simulink model "SF101A_MotQuadDetn"  (R2013b)
settings: Solver=FixedStepDiscrete  StartTime=0.0  StopTime=1  FixedStep=Ts  RelTol=1e-3
model workspace (MAT data in the model file):
  SLAMConfig_1_ATPP = [3707764736; 2; 1; 1; 1; 34]
values from neighbouring files (symbols this model uses):
  MotQuadDetnMotDirHysInsts = DataDict.Calibration    [SF101A_MotQuadDetn_DataDict.m]
  MOTTQCMDTOLR_MOTNWTMTR_F32 = DataDict.Constant    [SF101A_MotQuadDetn_DataDict.m]
undefined symbols (not defined in the file or in its folder): MotQuad1
libraries: simulink x5, NxtrAbslt x2, NxtrSign x2
(part 1 of 2)
settings Model: RecordCoverage=on  Creator=qzwc4r  LastModifiedBy=qzwc4r
settings DataIOCC: LimitDataPoints=off  SaveFormat=Structure  ReturnWorkspaceOutputs=on
settings OptimizationCC: BlockReduction=off  InlineParams=on  ZeroExternalMemoryAtStartup=off  ZeroInternalMemoryAtStartup=off  OptimizeModelRefInitCode=on  LifeSpan=1
settings DebuggingCC: SignalInfNanChecking=error  SignalRangeChecking=warning  UnderspecifiedInitializationDetection=Simplified  SolverPrmCheckMsg=error  InheritedTsInSrcMsg=error  DiscreteInheritContinuousMsg=error  SingleTaskRateTransMsg=error  TasksWithSamePriorityMsg=error  SigSpecEnsureSampleTimeMsg=error  CheckMatrixSingularityMsg=error  IntegerOverflowMsg=error  ParameterUnderflowMsg=error  ParameterPrecisionLossMsg=error  ParameterTunabilityLossMsg=error  FixptConstUnderflowMsg=warning  FixptConstOverflowMsg=warning  VectorMatrixConversionMsg=error  SignalLabelMismatchMsg=error  UnconnectedInputMsg=error  UnconnectedOutputMsg=error  UnconnectedLineMsg=error  SFcnCompatibilityMsg=error  UniqueDataStoreMsg=warning  BusObjectLabelMismatch=error  RootOutportRequireBusObject=error  AssertControl=DisableAll  ModelReferenceIOMsg=error  ModelReferenceVersionMismatchMessage=warning  ModelReferenceIOMismatchMessage=error  ModelReferenceCSMismatchMessage=warning  ModelReferenceDataLoggingMessage=error  StateNameClashWarn=warning  StrictBusMsg=ErrorOnBusTreatedAsVector  NonBusSignalsTreatedAsBus=error  SFUnexpectedBacktrackingDiag=error  SFInvalidInputDataAccessInChartInitDiag=error  SFNoUnconditionalDefaultTransitionDiag=error  SFTransitionOutsideNaturalParentDiag=error  SFUnconditionalTransitionShadowingDiag=error  SFUndirectedBroadcastEventsDiag=error
settings ModelReferenceCC: ModelReferenceNumInstancesAllowed=Single
settings RTWCC: SystemTargetFile=autosar.tlc  GenCodeOnly=on  TemplateMakefile=ert_default_tmf  Description=AUTOSAR  GenerateReport=on  ProcessScript=autosar_make_rtw_hook  LaunchReport=on
settings CodeAppCC: GenerateComments=off  IgnoreCustomStorageClasses=off  CustomSymbolStrType=$N$R$M  CustomSymbolStrBlkIO=$N$M  SimulinkBlockComments=off
settings STFCustomTargetCC: ParMdlRefBuildCompliant=on  CompOptLevelCompliant=on  IncludeMdlTerminateFcn=off  CombineOutputUpdateFcns=on  SuppressErrorStatus=on  ERTFirstTimeCompliant=on  ERTCustomFileBanners=on  SupportNonFinite=off  SupportComplex=off  SupportContinuousTime=off  SupportNonInlinedSFcns=off  MATLABClassNameForMDSCustomization=Simulink.SoftwareTarget.ERTCustomization  AutosarCompliant=on  GRTInterface=off  SystemTargetFile=autosar.tlc
settings ERTTargetCC: CodeReplacementLibrary=ANSI_C  ConcurrentExecutionCompliant=off  IncludeMdlTerminateFcn=off  SuppressErrorStatus=on  SupportNonFinite=off  SupportComplex=off  ModelStepFunctionPrototypeControlCompliant=off  CPPClassGenCompliant=off  AutosarCompliant=on  InlinedParameterPlacement=NonHierarchical  ERTCustomFileTemplate=example_file_process.tlc  EnableUserReplacementTypes=on

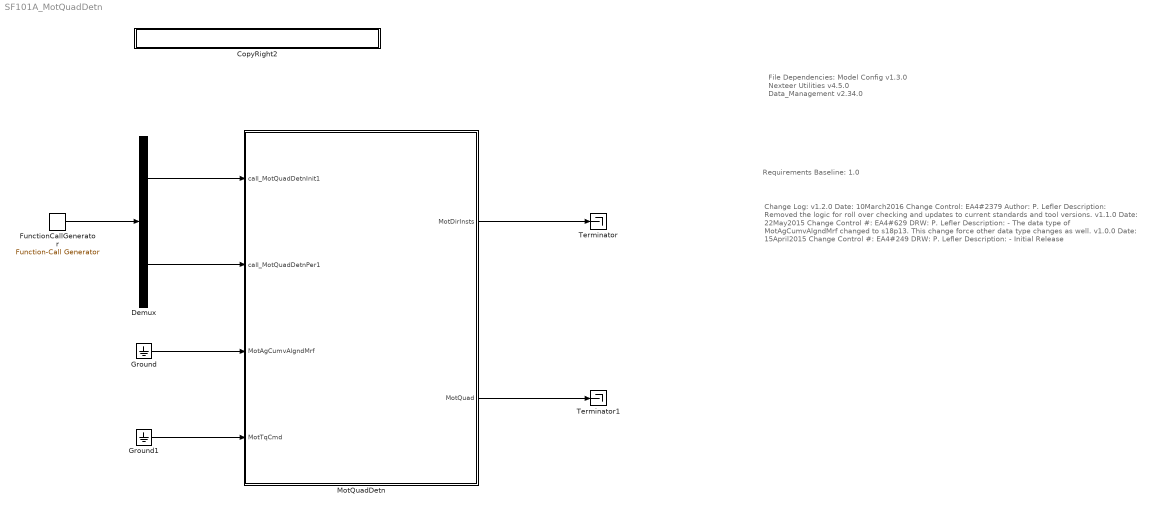
== system SF101A_MotQuadDetn ==
  note: File Dependencies:
      |
      | Model Config v1.3.0
      | Nexteer Utilities v4.5.0
      | Data_Management v2.34.0
  note: Requirements Baseline: 1.0
  note: Change Log:
      |
      | v1.2.0
      | Date: 10March2016
      | Change Control: EA4#2379
      | Author: P. Lefler
      | Description:
      | Removed the logic for roll over checking and updates to current standards and tool versions.
      |
      | v1.1.0
      | Date: 22May2015
      | Change Control #: EA4#629
      | DRW: P. Lefler
      | Description:
      | - The data type of MotAgCumvAlgndMrf changed to s18p13.
      |   This change force other data type changes as well.
      |
      | v1.0.0
      | Date: 15April2015
      | Change Control #: EA4#249
      | DRW: P. Lefler
      | Description:
      | - Initial Release
  CopyRight2 : Subsystem  Description=|  mask(Copyright Information){none=on}
      | Copyright info block.                                               
      |                                                                     
      | Place copyright information at the top of every subsystem in design.
      mask prompts: none "No parameters"
      mask help: Place copyright information at the top of every subsystem in design.
      mask Display:
      | NxtrConf = 'Nexteer Confidential';
      | 
      | sys = bdroot; %handle for the current model ("system")
      | first = get_param(sys,'Created');
      | if(isempty(first))
      |     first = datestr(now,'yyyy');
      | else
      |     first = first(end-3:end);  %year is last four digits
      | end
      | 
      | last = get_param(sys,'LastModifiedDate');
      | if isempty(last)
      |     last = datestr(now,'yyyy');
      | else
      |     last = last(end-3:end);
      | end
      | 
      | if strcmp(first,last)
      |     fprintf('%s -- Copyright %s Nexteer',NxtrConf,first)
      | else
      |     fprintf('%s -- %s%s- %s Nexteer',NxtrConf,char(169),first,last)
      | end
  Demux : Demux  Outputs=2
  FunctionCallGenerator : simulink/Ports & Subsystems/Function-Call Generator  RequirementInfo="{'linktype_rmi_doors' '0000bb40 (/E-STEER Core/SubSystem Specifications/Application Functions/SF99/SF101A Motor Quadrant Detection)' '#SF101A_63' 'true' 'REQ:  SF101A_63' '' } %GIDa_ba4b940a_c476_4c12_9873_433c070b2edb"  sample_time=0.002  numberOfIterations=1
  Ground : Ground
  Ground1 : Ground
  MotQuadDetn : Subsystem
  Terminator : Terminator
  Terminator1 : Terminator
  wires:
  Demux/1 -> MotQuadDetn/1(call_MotQuadDetnInit1)
  Demux/2 -> MotQuadDetn/2(call_MotQuadDetnPer1)
  FunctionCallGenerator/1 -> Demux/1
  Ground/1 -> MotQuadDetn/3(MotAgCumvAlgndMrf)
  MotQuadDetn/1(MotDirInsts) -> Terminator/1
  MotQuadDetn/2(MotQuad) -> Terminator1/1
  Ground1/1 -> MotQuadDetn/4(MotTqCmd)

== system SF101A_MotQuadDetn/CopyRight2 ==

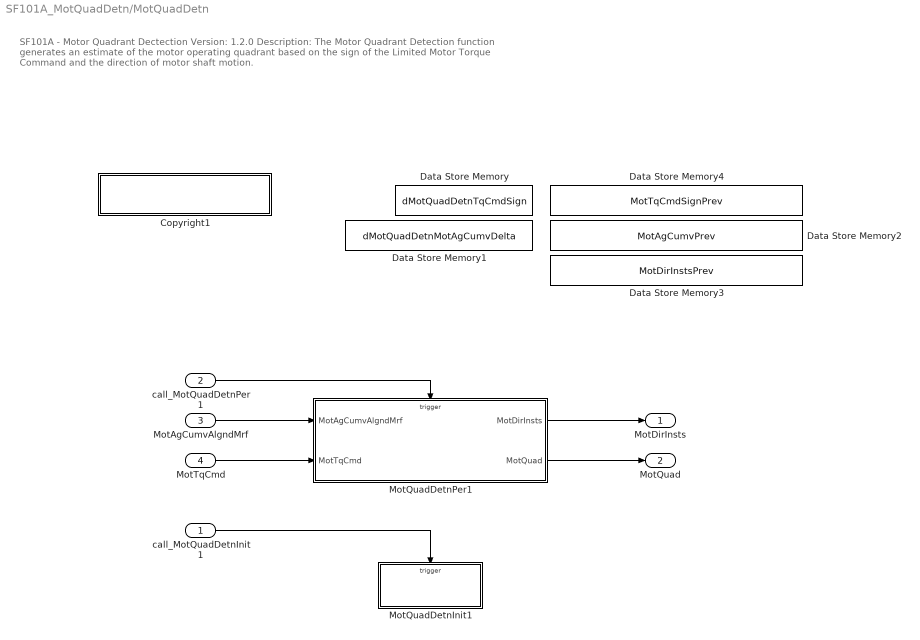
== system SF101A_MotQuadDetn/MotQuadDetn ==
  note: SF101A - Motor Quadrant Dectection
      | Version: 1.2.0
      | Description:
      | The Motor Quadrant Detection function generates an estimate of the motor operating quadrant based on the sign of the Limited Motor Torque Command and the direction of motor shaft motion.
  call_MotQuadDetnInit1 : Inport
  call_MotQuadDetnPer1 : Inport  Port=2
  MotAgCumvAlgndMrf : Inport  RequirementInfo="{'linktype_rmi_doors' '0000bb40 (/E-STEER Core/SubSystem Specifications/Application Functions/SF99/SF101A Motor Quadrant Detection)' '#SF101A_27' 'true' 'REQ:  SF101A_27' '' } %GIDa_ce1f5992_a30b_4fb4_84ed_8bc9c57286df"  Port=3  OutDataTypeStr=int32  PortDimensions=1
  MotTqCmd : Inport  RequirementInfo="{'linktype_rmi_doors' '0000bb40 (/E-STEER Core/SubSystem Specifications/Application Functions/SF99/SF101A Motor Quadrant Detection)' '#SF101A_38' 'true' 'REQ:  SF101A_38' '' } %GIDa_55ad6957_dc0e_47dc_876d_670590d48796"  Port=4  OutDataTypeStr=single  PortDimensions=1
  Copyright1 : Subsystem  Description=|  mask(Copyright Information){none=on}
      | Copyright info block.                                               
      |                                                                     
      | Place copyright information at the top of every subsystem in design.
      mask prompts: none "No parameters"
      mask help: Place copyright information at the top of every subsystem in design.
      mask Display:
      | NxtrConf = 'Nexteer Confidential';
      | 
      | sys = bdroot; %handle for the current model ("system")
      | first = get_param(sys,'Created');
      | if(isempty(first))
      |     first = datestr(now,'yyyy');
      | else
      |     first = first(end-3:end);  %year is last four digits
      | end
      | 
      | last = get_param(sys,'LastModifiedDate');
      | if isempty(last)
      |     last = datestr(now,'yyyy');
      | else
      |     last = last(end-3:end);
      | end
      | 
      | if strcmp(first,last)
      |     fprintf('%s\nCopyright  %s Nexteer',NxtrConf,first);
      | else
      |     fprintf('%s\n%s%s-%s Nexteer',NxtrConf,char(169),first,last);
      | end
  Data Store Memory : DataStoreMemory  DataStoreName=dMotQuadDetnTqCmdSign  StateMustResolveToSignalObject=on
  Data Store Memory1 : DataStoreMemory  DataStoreName=dMotQuadDetnMotAgCumvDelta  StateMustResolveToSignalObject=on
  Data Store Memory2 : DataStoreMemory  DataStoreName=MotAgCumvPrev  StateMustResolveToSignalObject=on
  Data Store Memory3 : DataStoreMemory  DataStoreName=MotDirInstsPrev  StateMustResolveToSignalObject=on
  Data Store Memory4 : DataStoreMemory  DataStoreName=MotTqCmdSignPrev  StateMustResolveToSignalObject=on
  MotQuadDetnInit1 : Subsystem  TreatAsAtomicUnit=on
  MotQuadDetnPer1 : Subsystem
  MotDirInsts : Outport  RequirementInfo="{'linktype_rmi_doors' '0000bb40 (/E-STEER Core/SubSystem Specifications/Application Functions/SF99/SF101A Motor Quadrant Detection)' '#SF101A_28' 'true' 'REQ:  SF101A_28' '' } %GIDa_c93875f8_cc59_405f_b59a_8f59cf744667"  OutDataTypeStr=int8  PortDimensions=1
  MotQuad : Outport  RequirementInfo="{'linktype_rmi_doors' '0000bb40 (/E-STEER Core/SubSystem Specifications/Application Functions/SF99/SF101A Motor Quadrant Detection)' '#SF101A_39' 'true' 'REQ:  SF101A_39' '' } %GIDa_9a3fad06_e616_455b_a302_26a30b94c3d7"  Port=2  OutDataTypeStr=Enum: MotQuad1  PortDimensions=1
  wires:
  MotQuadDetnPer1/2(MotQuad) -> MotQuad/1
  MotQuadDetnPer1/1(MotDirInsts) -> MotDirInsts/1
  MotTqCmd/1 -> MotQuadDetnPer1/2(MotTqCmd)
  MotAgCumvAlgndMrf/1 -> MotQuadDetnPer1/1(MotAgCumvAlgndMrf)
  call_MotQuadDetnPer1/1 -> MotQuadDetnPer1/Trigger
  call_MotQuadDetnInit1/1 -> MotQuadDetnInit1/Trigger

== system SF101A_MotQuadDetn/MotQuadDetn/Copyright1 ==

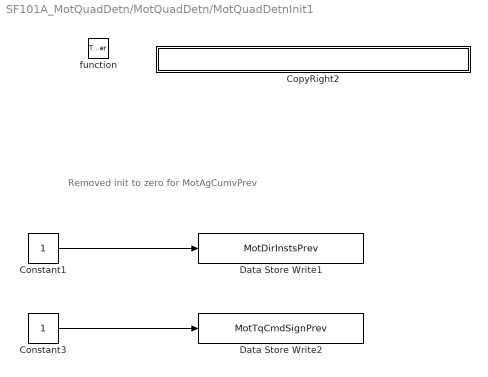
== system SF101A_MotQuadDetn/MotQuadDetn/MotQuadDetnInit1 ==
  note: Removed init to zero for MotAgCumvPrev
  function : TriggerPort  TriggerType=function-call
  Constant1 : Constant  RequirementInfo="{'linktype_rmi_doors' '0000bb40 (/E-STEER Core/SubSystem Specifications/Application Functions/SF99/SF101A Motor Quadrant Detection)' '#SF101A_49' 'true' 'REQ:  SF101A_49' '' } %GIDa_5d2ddbe5_3095_4ce2_977e_d4f70d111454"  OutDataTypeStr=int8
  Constant3 : Constant  RequirementInfo="{'linktype_rmi_doors' '0000bb40 (/E-STEER Core/SubSystem Specifications/Application Functions/SF99/SF101A Motor Quadrant Detection)' '#SF101A_55' 'true' 'REQ:  SF101A_55' '' } %GIDa_37157d88_6289_46d7_8e4c_5fdd13e4fc16"  OutDataTypeStr=int8
  CopyRight2 : Subsystem  Description=|  mask(Copyright Information){none=on}
      | Copyright info block.                                               
      |                                                                     
      | Place copyright information at the top of every subsystem in design.
      mask prompts: none "No parameters"
      mask help: Place copyright information at the top of every subsystem in design.
      mask Display:
      | NxtrConf = 'Nexteer Confidential';
      | 
      | sys = bdroot; %handle for the current model ("system")
      | first = get_param(sys,'Created');
      | if(isempty(first))
      |     first = datestr(now,'yyyy');
      | else
      |     first = first(end-3:end);  %year is last four digits
      | end
      | 
      | last = get_param(sys,'LastModifiedDate');
      | if isempty(last)
      |     last = datestr(now,'yyyy');
      | else
      |     last = last(end-3:end);
      | end
      | 
      | if strcmp(first,last)
      |     fprintf('%s -- Copyright %s Nexteer',NxtrConf,first)
      | else
      |     fprintf('%s -- %s%s- %s Nexteer',NxtrConf,char(169),first,last)
      | end
  Data Store Write1 : DataStoreWrite  RequirementInfo="{'linktype_rmi_doors' '0000bb40 (/E-STEER Core/SubSystem Specifications/Application Functions/SF99/SF101A Motor Quadrant Detection)' '#SF101A_49' 'true' 'REQ:  SF101A_49' '' } %GIDa_33825ee6_1fe0_4111_9478_8621974325d7"  DataStoreName=MotDirInstsPrev
  Data Store Write2 : DataStoreWrite  RequirementInfo="{'linktype_rmi_doors' '0000bb40 (/E-STEER Core/SubSystem Specifications/Application Functions/SF99/SF101A Motor Quadrant Detection)' '#SF101A_55' 'true' 'REQ:  SF101A_55' '' } %GIDa_0551e2d3_8a0f_49e4_ae02_6b9d57023870"  DataStoreName=MotTqCmdSignPrev
  wires:
  Constant1/1 -> Data Store Write1/1
  Constant3/1 -> Data Store Write2/1

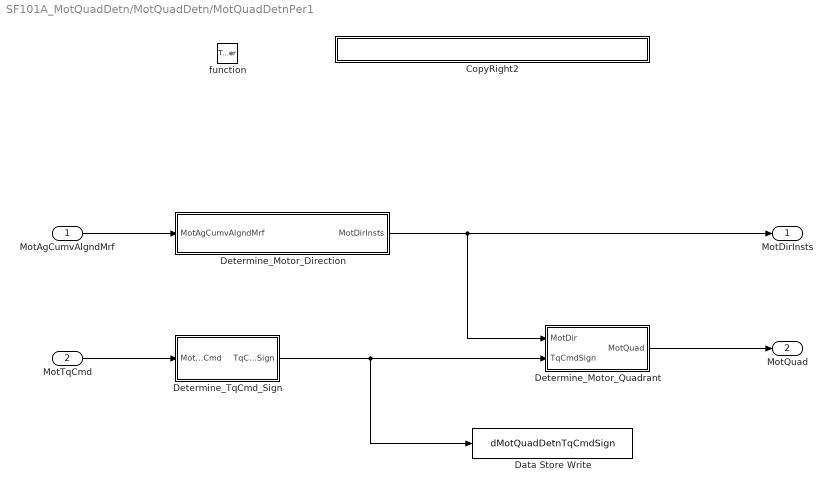
== system SF101A_MotQuadDetn/MotQuadDetn/MotQuadDetnPer1 ==
  MotAgCumvAlgndMrf : Inport  OutDataTypeStr=int32  PortDimensions=1
  MotTqCmd : Inport  Port=2  OutDataTypeStr=single  PortDimensions=1
  function : TriggerPort  TriggerType=function-call  PortDimensions=1
  CopyRight2 : Subsystem  Description=|  mask(Copyright Information){none=on}
      | Copyright info block.                                               
      |                                                                     
      | Place copyright information at the top of every subsystem in design.
      mask prompts: none "No parameters"
      mask help: Place copyright information at the top of every subsystem in design.
      mask Display:
      | NxtrConf = 'Nexteer Confidential';
      | 
      | sys = bdroot; %handle for the current model ("system")
      | first = get_param(sys,'Created');
      | if(isempty(first))
      |     first = datestr(now,'yyyy');
      | else
      |     first = first(end-3:end);  %year is last four digits
      | end
      | 
      | last = get_param(sys,'LastModifiedDate');
      | if isempty(last)
      |     last = datestr(now,'yyyy');
      | else
      |     last = last(end-3:end);
      | end
      | 
      | if strcmp(first,last)
      |     fprintf('%s -- Copyright %s Nexteer',NxtrConf,first)
      | else
      |     fprintf('%s -- %s%s- %s Nexteer',NxtrConf,char(169),first,last)
      | end
  Data Store Write : DataStoreWrite  DataStoreName=dMotQuadDetnTqCmdSign
  Determine_Motor_Direction : Subsystem  TreatAsAtomicUnit=on
  Determine_Motor_Quadrant : Subsystem  RequirementInfo="{'linktype_rmi_doors' '0000bb40 (/E-STEER Core/SubSystem Specifications/Application Functions/SF99/SF101A Motor Quadrant Detection)' '#SF101A_53' 'true' 'REQ:  SF101A_53' '' } %GIDa_02fb40bd_96d0_49ba_b5f0_97be253398e5"  TreatAsAtomicUnit=on
  Determine_TqCmd_Sign : Subsystem  RequirementInfo="{'linktype_rmi_doors' '0000bb40 (/E-STEER Core/SubSystem Specifications/Application Functions/SF99/SF101A Motor Quadrant Detection)' '#SF101A_51' 'true' 'REQ:  SF101A_51' '' } %GIDa_eb9f9e8f_fed9_4594_8edb_e305cda2f43b"  TreatAsAtomicUnit=on
  MotDirInsts : Outport  OutDataTypeStr=int8  PortDimensions=1
  MotQuad : Outport  Port=2  OutDataTypeStr=Enum: MotQuad1  PortDimensions=1
  wires:
  MotAgCumvAlgndMrf/1 -> Determine_Motor_Direction/1(MotAgCumvAlgndMrf)
  MotTqCmd/1 -> Determine_TqCmd_Sign/1(MotTqCmd)
  Determine_TqCmd_Sign/1(TqCmdSign) -> Data Store Write/1, Determine_Motor_Quadrant/2(TqCmdSign)
  Determine_Motor_Quadrant/1(MotQuad) -> MotQuad/1
  Determine_Motor_Direction/1(MotDirInsts) -> MotDirInsts/1, Determine_Motor_Quadrant/1(MotDir)

== system SF101A_MotQuadDetn/MotQuadDetn/MotQuadDetnInit1/CopyRight2 ==

== system SF101A_MotQuadDetn/MotQuadDetn/MotQuadDetnPer1/CopyRight2 ==

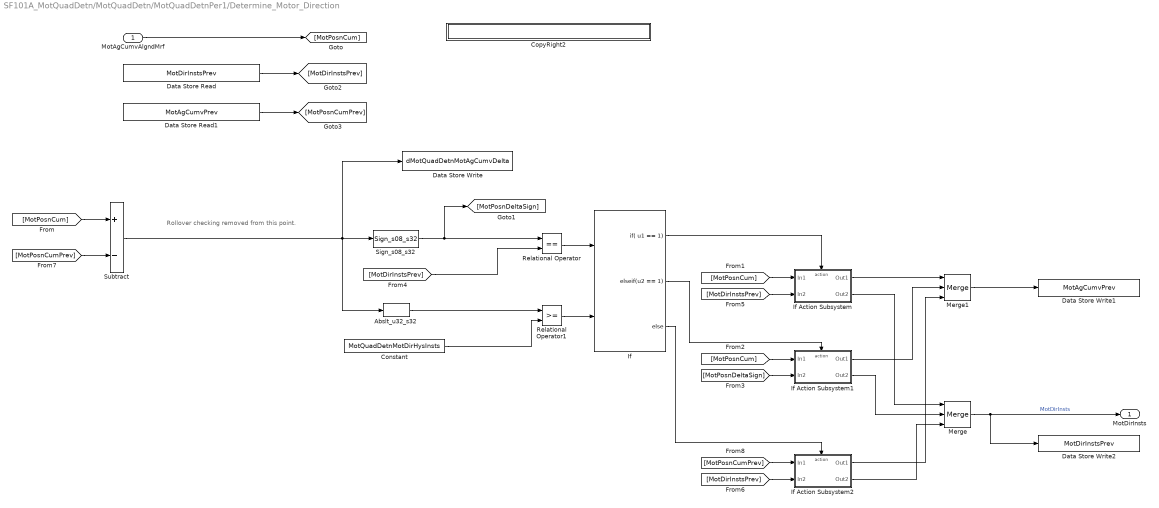
== system SF101A_MotQuadDetn/MotQuadDetn/MotQuadDetnPer1/Determine_Motor_Direction ==
  note: Rollover checking removed from this point.
  MotAgCumvAlgndMrf : Inport  RequirementInfo="{'linktype_rmi_doors' '0000bb40 (/E-STEER Core/SubSystem Specifications/Application Functions/SF99/SF101A Motor Quadrant Detection)' '#SF101A_46' 'true' 'REQ:  SF101A_46' '' ; 'linktype_rmi_doors' '0000bb40 (/E-STEER Core/SubSystem Specifications/Application Functions/SF99/SF101A Motor Quadrant Detection)' '#SF101A_44' 'true' 'REQ:  SF101A_44' '' } %GIDa_33168858_7d05_4f18_8f4c_06695088646f"
  Abslt_u32_s32 : NxtrAbslt/Abslt_u32_s32  RequirementInfo="{'linktype_rmi_doors' '0000bb40 (/E-STEER Core/SubSystem Specifications/Application Functions/SF99/SF101A Motor Quadrant Detection)' '#SF101A_47' 'true' 'REQ:  SF101A_47' '' } %GIDa_46c42c72_ca25_40ef_8955_407cadf23955"  SFunctionSpec=uint32 y1 = Abslt_u32_s32( int32 u1)
      settings: AttributesFormatString=%<Name>
  Constant : Constant  RequirementInfo="{'linktype_rmi_doors' '0000bb40 (/E-STEER Core/SubSystem Specifications/Application Functions/SF99/SF101A Motor Quadrant Detection)' '#SF101A_47' 'true' 'REQ:  SF101A_47' '' } %GIDa_7af5e37b_1e32_4084_9345_8c4ddd29f877"  Value=MotQuadDetnMotDirHysInsts
  CopyRight2 : Subsystem  Description=|  mask(Copyright Information){none=on}
      | Copyright info block.                                               
      |                                                                     
      | Place copyright information at the top of every subsystem in design.
      mask prompts: none "No parameters"
      mask help: Place copyright information at the top of every subsystem in design.
      mask Display:
      | NxtrConf = 'Nexteer Confidential';
      | 
      | sys = bdroot; %handle for the current model ("system")
      | first = get_param(sys,'Created');
      | if(isempty(first))
      |     first = datestr(now,'yyyy');
      | else
      |     first = first(end-3:end);  %year is last four digits
      | end
      | 
      | last = get_param(sys,'LastModifiedDate');
      | if isempty(last)
      |     last = datestr(now,'yyyy');
      | else
      |     last = last(end-3:end);
      | end
      | 
      | if strcmp(first,last)
      |     fprintf('%s -- Copyright %s Nexteer',NxtrConf,first)
      | else
      |     fprintf('%s -- %s%s- %s Nexteer',NxtrConf,char(169),first,last)
      | end
  Data Store Read : DataStoreRead  DataStoreName=MotDirInstsPrev
  Data Store Read1 : DataStoreRead  RequirementInfo="{'linktype_rmi_doors' '0000bb40 (/E-STEER Core/SubSystem Specifications/Application Functions/SF99/SF101A Motor Quadrant Detection)' '#SF101A_46' 'true' 'REQ:  SF101A_46' '' ; 'linktype_rmi_doors' '0000bb40 (/E-STEER Core/SubSystem Specifications/Application Functions/SF99/SF101A Motor Quadrant Detection)' '#SF101A_44' 'true' 'REQ:  SF101A_44' '' } %GIDa_269066c3_13eb_447a_8e55_95ebd7583ac8"  DataStoreName=MotAgCumvPrev
  Data Store Write : DataStoreWrite  DataStoreName=dMotQuadDetnMotAgCumvDelta
  Data Store Write1 : DataStoreWrite  RequirementInfo="{'linktype_rmi_doors' '0000bb40 (/E-STEER Core/SubSystem Specifications/Application Functions/SF99/SF101A Motor Quadrant Detection)' '#SF101A_46' 'true' 'REQ:  SF101A_46' '' ; 'linktype_rmi_doors' '0000bb40 (/E-STEER Core/SubSystem Specifications/Application Functions/SF99/SF101A Motor Quadrant Detection)' '#SF101A_44' 'true' 'REQ:  SF101A_44' '' } %GIDa_9bff677e_e394_40d8_a69c_2132827397bf"  DataStoreName=MotAgCumvPrev
  Data Store Write2 : DataStoreWrite  DataStoreName=MotDirInstsPrev
  If : If  NumInputs=2  IfExpression=u1 == 1  ElseIfExpressions=u2 == 1
  If Action Subsystem : Subsystem  TreatAsAtomicUnit=on
      settings: RTWSystemCode=Inline
  If Action Subsystem1 : Subsystem  TreatAsAtomicUnit=on
      settings: RTWSystemCode=Inline
  If Action Subsystem2 : Subsystem  TreatAsAtomicUnit=on
      settings: RTWSystemCode=Inline
  Merge : Merge  Inputs=3
  Merge1 : Merge  Inputs=3
  Relational Operator : RelationalOperator  Operator===  OutDataTypeStr=boolean
  Relational Operator1 : RelationalOperator  OutDataTypeStr=boolean
  Sign_s08_s32 : NxtrSign/Sign_s08_s32  RequirementInfo="{'linktype_rmi_doors' '0000bb40 (/E-STEER Core/SubSystem Specifications/Application Functions/SF99/SF101A Motor Quadrant Detection)' '#SF101A_44' 'true' 'REQ:  SF101A_44' '' ; 'linktype_rmi_doors' '0000bb40 (/E-STEER Core/SubSystem Specifications/Application Functions/SF99/SF101A Motor Quadrant Detection)' '#SF101A_57' 'true' 'REQ:  SF101A_57' '' } %GIDa_4174577c_cdf4_4d25_8cc3_032965890b4a"  SFunctionSpec=int8 y1 = Sign_s08_s32( int32 u1)
  Subtract : Sum  RequirementInfo="{'linktype_rmi_doors' '0000bb40 (/E-STEER Core/SubSystem Specifications/Application Functions/SF99/SF101A Motor Quadrant Detection)' '#SF101A_46' 'true' 'REQ:  SF101A_46' '' ; 'linktype_rmi_doors' '0000bb40 (/E-STEER Core/SubSystem Specifications/Application Functions/SF99/SF101A Motor Quadrant Detection)' '#SF101A_44' 'true' 'REQ:  SF101A_44' '' } %GIDa_5fce257d_7301_4941_b31f_c4ddb6e8cb64"  Inputs=+-
  MotDirInsts : Outport
  wires:
  [MotPosnCumPrev] -> Subtract/2
  Sign_s08_s32/1 -> Relational Operator/1, [MotPosnDeltaSign]
  If/1 -> If Action Subsystem/Action
  If/2 -> If Action Subsystem1/Action
  MotAgCumvAlgndMrf/1 -> [MotPosnCum]
  [MotPosnCum] -> Subtract/1
  [MotPosnCum] -> If Action Subsystem/1(In1)
  [MotPosnCum] -> If Action Subsystem1/1(In1)
  [MotPosnDeltaSign] -> If Action Subsystem1/2(In2)
  [MotDirInstsPrev] -> Relational Operator/2
  [MotPosnCumPrev] -> If Action Subsystem2/1(In1)
  If/3 -> If Action Subsystem2/Action
  If Action Subsystem2/2(Out2) -> Merge/3
  If Action Subsystem1/2(Out2) -> Merge/2
  If Action Subsystem/2(Out2) -> Merge/1
  Merge/1 -> Data Store Write2/1, MotDirInsts/1  "MotDirInsts"
  If Action Subsystem/1(Out1) -> Merge1/1
  If Action Subsystem1/1(Out1) -> Merge1/2
  If Action Subsystem2/1(Out1) -> Merge1/3
  Merge1/1 -> Data Store Write1/1
  Subtract/1 -> Data Store Write/1, Abslt_u32_s32/1, Sign_s08_s32/1
  [MotDirInstsPrev] -> If Action Subsystem/2(In2)
  [MotDirInstsPrev] -> If Action Subsystem2/2(In2)
  Data Store Read/1 -> [MotDirInstsPrev]
  Data Store Read1/1 -> [MotPosnCumPrev]
  Constant/1 -> Relational Operator1/2
  Abslt_u32_s32/1 -> Relational Operator1/1
  Relational Operator1/1 -> If/2
  Relational Operator/1 -> If/1

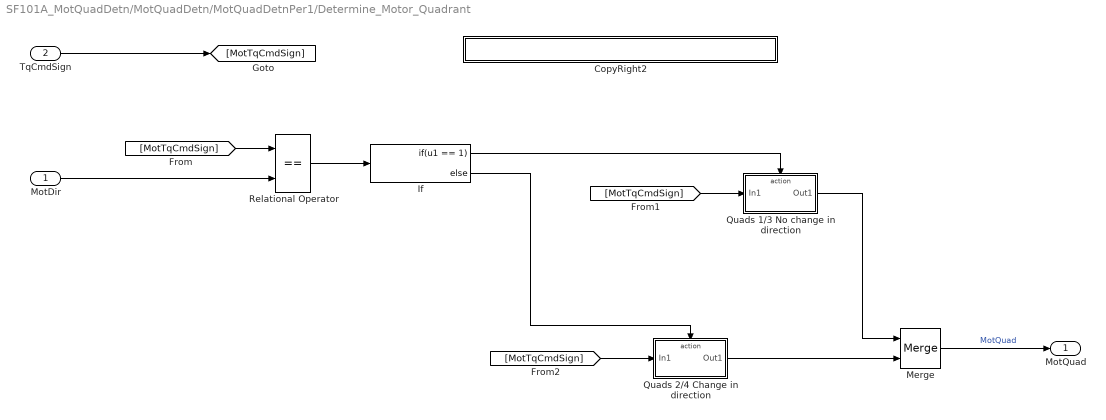
== system SF101A_MotQuadDetn/MotQuadDetn/MotQuadDetnPer1/Determine_Motor_Quadrant ==
  MotDir : Inport
  TqCmdSign : Inport  Port=2
  CopyRight2 : Subsystem  Description=|  mask(Copyright Information){none=on}
      | Copyright info block.                                               
      |                                                                     
      | Place copyright information at the top of every subsystem in design.
      mask prompts: none "No parameters"
      mask help: Place copyright information at the top of every subsystem in design.
      mask Display:
      | NxtrConf = 'Nexteer Confidential';
      | 
      | sys = bdroot; %handle for the current model ("system")
      | first = get_param(sys,'Created');
      | if(isempty(first))
      |     first = datestr(now,'yyyy');
      | else
      |     first = first(end-3:end);  %year is last four digits
      | end
      | 
      | last = get_param(sys,'LastModifiedDate');
      | if isempty(last)
      |     last = datestr(now,'yyyy');
      | else
      |     last = last(end-3:end);
      | end
      | 
      | if strcmp(first,last)
      |     fprintf('%s -- Copyright %s Nexteer',NxtrConf,first)
      | else
      |     fprintf('%s -- %s%s- %s Nexteer',NxtrConf,char(169),first,last)
      | end
  If : If  RequirementInfo="{'linktype_rmi_doors' '0000bb40 (/E-STEER Core/SubSystem Specifications/Application Functions/SF99/SF101A Motor Quadrant Detection)' '#SF101A_54' 'true' 'REQ:  SF101A_54' '' } %GIDa_7ecc17ff_8f5e_4b14_8da8_ae67d5ff9ccc"  IfExpression=u1 == 1
  Merge : Merge  RequirementInfo="{'linktype_rmi_doors' '0000bb40 (/E-STEER Core/SubSystem Specifications/Application Functions/SF99/SF101A Motor Quadrant Detection)' '#SF101A_54' 'true' 'REQ:  SF101A_54' '' } %GIDa_c93a8099_e8e5_4c0b_987a_8154384b51c5"
  Quads 1/3 No change in direction : Subsystem  RequirementInfo="{'linktype_rmi_doors' '0000bb40 (/E-STEER Core/SubSystem Specifications/Application Functions/SF99/SF101A Motor Quadrant Detection)' '#SF101A_54' 'true' 'REQ:  SF101A_54' '' } %GIDa_1c85d6fb_bcbe_4ead_8f35_8795b5e2ff89"  TreatAsAtomicUnit=on
      settings: RTWSystemCode=Inline
  Quads 2/4 Change in direction : Subsystem  RequirementInfo="{'linktype_rmi_doors' '0000bb40 (/E-STEER Core/SubSystem Specifications/Application Functions/SF99/SF101A Motor Quadrant Detection)' '#SF101A_54' 'true' 'REQ:  SF101A_54' '' } %GIDa_e2a8a1e9_6f7b_4770_8502_8c1a72a8d8f8"  TreatAsAtomicUnit=on
      settings: RTWSystemCode=Inline
  Relational Operator : RelationalOperator  RequirementInfo="{'linktype_rmi_doors' '0000bb40 (/E-STEER Core/SubSystem Specifications/Application Functions/SF99/SF101A Motor Quadrant Detection)' '#SF101A_54' 'true' 'REQ:  SF101A_54' '' } %GIDa_b4a959e3_569f_4f7a_bb72_55e412dce501"  Operator===  OutDataTypeStr=boolean
  MotQuad : Outport
  wires:
  Relational Operator/1 -> If/1
  If/1 -> Quads 1/3 No change in direction/Action
  If/2 -> Quads 2/4 Change in direction/Action
  [MotTqCmdSign] -> Relational Operator/1
  [MotTqCmdSign] -> Quads 1/3 No change in direction/1(In1)
  [MotTqCmdSign] -> Quads 2/4 Change in direction/1(In1)
  Quads 2/4 Change in direction/1(Out1) -> Merge/2
  Quads 1/3 No change in direction/1(Out1) -> Merge/1
  Merge/1 -> MotQuad/1  "MotQuad"
  MotDir/1 -> Relational Operator/2
  TqCmdSign/1 -> [MotTqCmdSign]

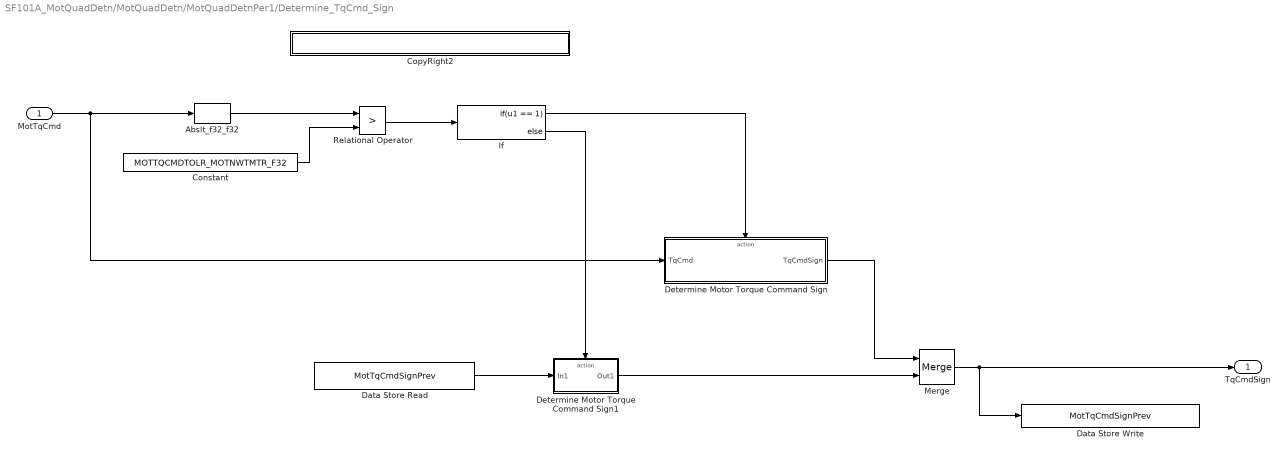
== system SF101A_MotQuadDetn/MotQuadDetn/MotQuadDetnPer1/Determine_TqCmd_Sign ==
  MotTqCmd : Inport
  Abslt_f32_f32 : NxtrAbslt/Abslt_f32_f32  RequirementInfo="{'linktype_rmi_doors' '0000bb40 (/E-STEER Core/SubSystem Specifications/Application Functions/SF99/SF101A Motor Quadrant Detection)' '#SF101A_51' 'true' 'REQ:  SF101A_51' '' ; 'linktype_rmi_doors' '0000bb40 (/E-STEER Core/SubSystem Specifications/Application Functions/SF99/SF101A Motor Quadrant Detection)' '#SF101A_52' 'true' 'REQ:  SF101A_52' '' } %GIDa_f90e4f93_60c7_4e66_b13a_2d2178dfe548"  SFunctionSpec=single y1 = Abslt_f32_f32(single u1)
      settings: AttributesFormatString=%<Name>
  Constant : Constant  RequirementInfo="{'linktype_rmi_doors' '0000bb40 (/E-STEER Core/SubSystem Specifications/Application Functions/SF99/SF101A Motor Quadrant Detection)' '#SF101A_51' 'true' 'REQ:  SF101A_51' '' ; 'linktype_rmi_doors' '0000bb40 (/E-STEER Core/SubSystem Specifications/Application Functions/SF99/SF101A Motor Quadrant Detection)' '#SF101A_52' 'true' 'REQ:  SF101A_52' '' } %GIDa_e193f212_06fe_40ea_a857_e74bcfb91209"  Value=MOTTQCMDTOLR_MOTNWTMTR_F32
  CopyRight2 : Subsystem  Description=|  mask(Copyright Information){none=on}
      | Copyright info block.                                               
      |                                                                     
      | Place copyright information at the top of every subsystem in design.
      mask prompts: none "No parameters"
      mask help: Place copyright information at the top of every subsystem in design.
      mask Display:
      | NxtrConf = 'Nexteer Confidential';
      | 
      | sys = bdroot; %handle for the current model ("system")
      | first = get_param(sys,'Created');
      | if(isempty(first))
      |     first = datestr(now,'yyyy');
      | else
      |     first = first(end-3:end);  %year is last four digits
      | end
      | 
      | last = get_param(sys,'LastModifiedDate');
      | if isempty(last)
      |     last = datestr(now,'yyyy');
      | else
      |     last = last(end-3:end);
      | end
      | 
      | if strcmp(first,last)
      |     fprintf('%s -- Copyright %s Nexteer',NxtrConf,first)
      | else
      |     fprintf('%s -- %s%s- %s Nexteer',NxtrConf,char(169),first,last)
      | end
  Data Store Read : DataStoreRead  RequirementInfo="{'linktype_rmi_doors' '0000bb40 (/E-STEER Core/SubSystem Specifications/Application Functions/SF99/SF101A Motor Quadrant Detection)' '#SF101A_51' 'true' 'REQ:  SF101A_51' '' ; 'linktype_rmi_doors' '0000bb40 (/E-STEER Core/SubSystem Specifications/Application Functions/SF99/SF101A Motor Quadrant Detection)' '#SF101A_52' 'true' 'REQ:  SF101A_52' '' } %GIDa_78055383_fd33_4f32_a792_942b06857283"  DataStoreName=MotTqCmdSignPrev
  Data Store Write : DataStoreWrite  RequirementInfo="{'linktype_rmi_doors' '0000bb40 (/E-STEER Core/SubSystem Specifications/Application Functions/SF99/SF101A Motor Quadrant Detection)' '#SF101A_51' 'true' 'REQ:  SF101A_51' '' ; 'linktype_rmi_doors' '0000bb40 (/E-STEER Core/SubSystem Specifications/Application Functions/SF99/SF101A Motor Quadrant Detection)' '#SF101A_52' 'true' 'REQ:  SF101A_52' '' } %GIDa_24469eb5_099e_4038_8906_40b7feb2eb99"  DataStoreName=MotTqCmdSignPrev
  Determine Motor Torque Command Sign : Subsystem  RequirementInfo="{'linktype_rmi_doors' '0000bb40 (/E-STEER Core/SubSystem Specifications/Application Functions/SF99/SF101A Motor Quadrant Detection)' '#SF101A_51' 'true' 'REQ:  SF101A_51' '' ; 'linktype_rmi_doors' '0000bb40 (/E-STEER Core/SubSystem Specifications/Application Functions/SF99/SF101A Motor Quadrant Detection)' '#SF101A_52' 'true' 'REQ:  SF101A_52' '' } %GIDa_61fe0f43_522f_48ca_920e_c2c1a6f78d79"  TreatAsAtomicUnit=on
      settings: RTWSystemCode=Inline
  Determine Motor Torque Command Sign1 : Subsystem  RequirementInfo="{'linktype_rmi_doors' '0000bb40 (/E-STEER Core/SubSystem Specifications/Application Functions/SF99/SF101A Motor Quadrant Detection)' '#SF101A_51' 'true' 'REQ:  SF101A_51' '' ; 'linktype_rmi_doors' '0000bb40 (/E-STEER Core/SubSystem Specifications/Application Functions/SF99/SF101A Motor Quadrant Detection)' '#SF101A_52' 'true' 'REQ:  SF101A_52' '' } %GIDa_affc5b2e_15d5_4e89_95dc_cc5434e6cbe1"  TreatAsAtomicUnit=on
      settings: RTWSystemCode=Inline
  If : If  RequirementInfo="{'linktype_rmi_doors' '0000bb40 (/E-STEER Core/SubSystem Specifications/Application Functions/SF99/SF101A Motor Quadrant Detection)' '#SF101A_51' 'true' 'REQ:  SF101A_51' '' ; 'linktype_rmi_doors' '0000bb40 (/E-STEER Core/SubSystem Specifications/Application Functions/SF99/SF101A Motor Quadrant Detection)' '#SF101A_52' 'true' 'REQ:  SF101A_52' '' } %GIDa_88fa73d7_69aa_4ed8_a623_a64017565c6f"  IfExpression=u1 == 1
  Merge : Merge  RequirementInfo="{'linktype_rmi_doors' '0000bb40 (/E-STEER Core/SubSystem Specifications/Application Functions/SF99/SF101A Motor Quadrant Detection)' '#SF101A_51' 'true' 'REQ:  SF101A_51' '' ; 'linktype_rmi_doors' '0000bb40 (/E-STEER Core/SubSystem Specifications/Application Functions/SF99/SF101A Motor Quadrant Detection)' '#SF101A_52' 'true' 'REQ:  SF101A_52' '' } %GIDa_1ce0716b_fd82_435d_bb2b_74304127719f"
  Relational Operator : RelationalOperator  RequirementInfo="{'linktype_rmi_doors' '0000bb40 (/E-STEER Core/SubSystem Specifications/Application Functions/SF99/SF101A Motor Quadrant Detection)' '#SF101A_51' 'true' 'REQ:  SF101A_51' '' ; 'linktype_rmi_doors' '0000bb40 (/E-STEER Core/SubSystem Specifications/Application Functions/SF99/SF101A Motor Quadrant Detection)' '#SF101A_52' 'true' 'REQ:  SF101A_52' '' } %GIDa_b0ce9b17_668c_431a_a404_14e97e09b91d"  Operator=>  OutDataTypeStr=boolean
  TqCmdSign : Outport
  wires:
  MotTqCmd/1 -> Abslt_f32_f32/1, Determine Motor Torque Command Sign/1(TqCmd)
  Abslt_f32_f32/1 -> Relational Operator/1
  Constant/1 -> Relational Operator/2
  Relational Operator/1 -> If/1
  If/1 -> Determine Motor Torque Command Sign/Action
  If/2 -> Determine Motor Torque Command Sign1/Action
  Determine Motor Torque Command Sign1/1(Out1) -> Merge/2
  Merge/1 -> Data Store Write/1, TqCmdSign/1
  Data Store Read/1 -> Determine Motor Torque Command Sign1/1(In1)
  Determine Motor Torque Command Sign/1(TqCmdSign) -> Merge/1

== system SF101A_MotQuadDetn/MotQuadDetn/MotQuadDetnPer1/Determine_Motor_Direction/CopyRight2 ==

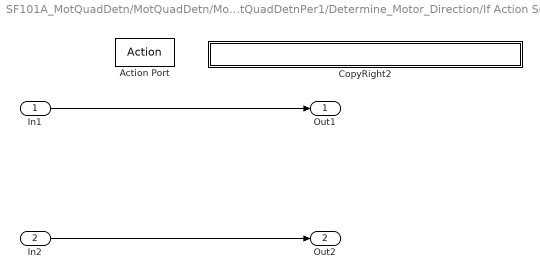
== system SF101A_MotQuadDetn/MotQuadDetn/MotQuadDetnPer1/Determine_Motor_Direction/If Action Subsystem ==
  In1 : Inport
  In2 : Inport  Port=2
  Action Port : ActionPort  ActionType=then
  CopyRight2 : Subsystem  Description=|  mask(Copyright Information){none=on}
      | Copyright info block.                                               
      |                                                                     
      | Place copyright information at the top of every subsystem in design.
      mask prompts: none "No parameters"
      mask help: Place copyright information at the top of every subsystem in design.
      mask Display:
      | NxtrConf = 'Nexteer Confidential';
      | 
      | sys = bdroot; %handle for the current model ("system")
      | first = get_param(sys,'Created');
      | if(isempty(first))
      |     first = datestr(now,'yyyy');
      | else
      |     first = first(end-3:end);  %year is last four digits
      | end
      | 
      | last = get_param(sys,'LastModifiedDate');
      | if isempty(last)
      |     last = datestr(now,'yyyy');
      | else
      |     last = last(end-3:end);
      | end
      | 
      | if strcmp(first,last)
      |     fprintf('%s -- Copyright %s Nexteer',NxtrConf,first)
      | else
      |     fprintf('%s -- %s%s- %s Nexteer',NxtrConf,char(169),first,last)
      | end
  Out1 : Outport
  Out2 : Outport  Port=2
  wires:
  In1/1 -> Out1/1
  In2/1 -> Out2/1

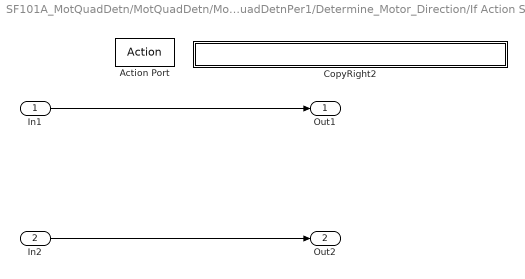
== system SF101A_MotQuadDetn/MotQuadDetn/MotQuadDetnPer1/Determine_Motor_Direction/If Action Subsystem1 ==
  In1 : Inport
  In2 : Inport  Port=2
  Action Port : ActionPort  ActionType=elseif
  CopyRight2 : Subsystem  Description=|  mask(Copyright Information){none=on}
      | Copyright info block.                                               
      |                                                                     
      | Place copyright information at the top of every subsystem in design.
      mask prompts: none "No parameters"
      mask help: Place copyright information at the top of every subsystem in design.
      mask Display:
      | NxtrConf = 'Nexteer Confidential';
      | 
      | sys = bdroot; %handle for the current model ("system")
      | first = get_param(sys,'Created');
      | if(isempty(first))
      |     first = datestr(now,'yyyy');
      | else
      |     first = first(end-3:end);  %year is last four digits
      | end
      | 
      | last = get_param(sys,'LastModifiedDate');
      | if isempty(last)
      |     last = datestr(now,'yyyy');
      | else
      |     last = last(end-3:end);
      | end
      | 
      | if strcmp(first,last)
      |     fprintf('%s -- Copyright %s Nexteer',NxtrConf,first)
      | else
      |     fprintf('%s -- %s%s- %s Nexteer',NxtrConf,char(169),first,last)
      | end
  Out1 : Outport
  Out2 : Outport  Port=2
  wires:
  In2/1 -> Out2/1
  In1/1 -> Out1/1

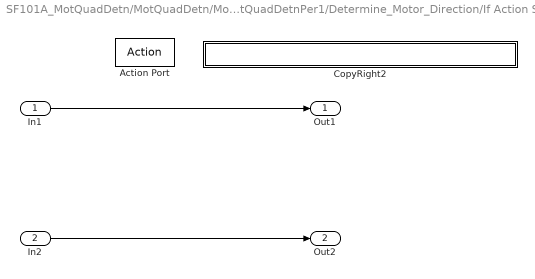
== system SF101A_MotQuadDetn/MotQuadDetn/MotQuadDetnPer1/Determine_Motor_Direction/If Action Subsystem2 ==
  In1 : Inport
  In2 : Inport  Port=2
  Action Port : ActionPort  ActionType=else
  CopyRight2 : Subsystem  Description=|  mask(Copyright Information){none=on}
      | Copyright info block.                                               
      |                                                                     
      | Place copyright information at the top of every subsystem in design.
      mask prompts: none "No parameters"
      mask help: Place copyright information at the top of every subsystem in design.
      mask Display:
      | NxtrConf = 'Nexteer Confidential';
      | 
      | sys = bdroot; %handle for the current model ("system")
      | first = get_param(sys,'Created');
      | if(isempty(first))
      |     first = datestr(now,'yyyy');
      | else
      |     first = first(end-3:end);  %year is last four digits
      | end
      | 
      | last = get_param(sys,'LastModifiedDate');
      | if isempty(last)
      |     last = datestr(now,'yyyy');
      | else
      |     last = last(end-3:end);
      | end
      | 
      | if strcmp(first,last)
      |     fprintf('%s -- Copyright %s Nexteer',NxtrConf,first)
      | else
      |     fprintf('%s -- %s%s- %s Nexteer',NxtrConf,char(169),first,last)
      | end
  Out1 : Outport
  Out2 : Outport  Port=2
  wires:
  In1/1 -> Out1/1
  In2/1 -> Out2/1

== system SF101A_MotQuadDetn/MotQuadDetn/MotQuadDetnPer1/Determine_Motor_Quadrant/CopyRight2 ==

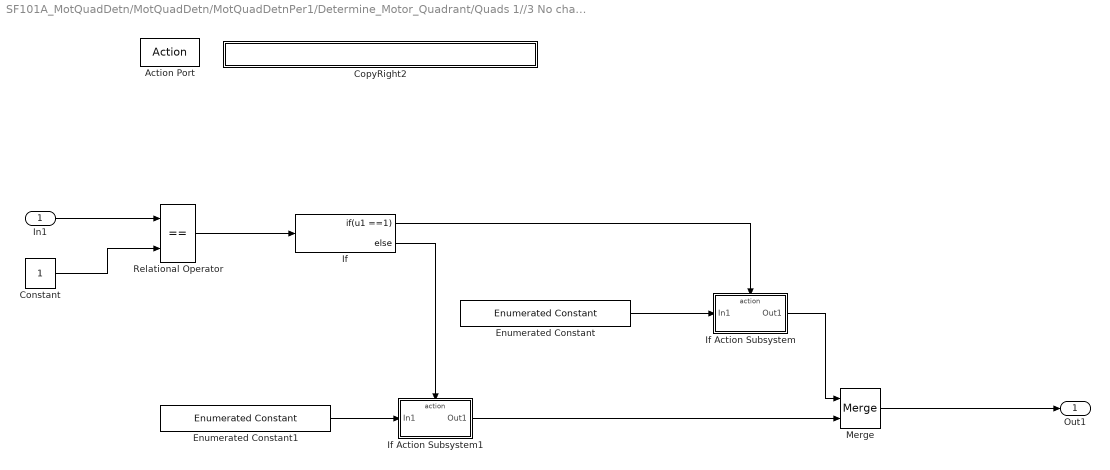
== system SF101A_MotQuadDetn/MotQuadDetn/MotQuadDetnPer1/Determine_Motor_Quadrant/Quads 1//3 No change in direction ==
  In1 : Inport
  Action Port : ActionPort  ActionType=then
  Constant : Constant  OutDataTypeStr=int8
  CopyRight2 : Subsystem  Description=|  mask(Copyright Information){none=on}
      | Copyright info block.                                               
      |                                                                     
      | Place copyright information at the top of every subsystem in design.
      mask prompts: none "No parameters"
      mask help: Place copyright information at the top of every subsystem in design.
      mask Display:
      | NxtrConf = 'Nexteer Confidential';
      | 
      | sys = bdroot; %handle for the current model ("system")
      | first = get_param(sys,'Created');
      | if(isempty(first))
      |     first = datestr(now,'yyyy');
      | else
      |     first = first(end-3:end);  %year is last four digits
      | end
      | 
      | last = get_param(sys,'LastModifiedDate');
      | if isempty(last)
      |     last = datestr(now,'yyyy');
      | else
      |     last = last(end-3:end);
      | end
      | 
      | if strcmp(first,last)
      |     fprintf('%s -- Copyright %s Nexteer',NxtrConf,first)
      | else
      |     fprintf('%s -- %s%s- %s Nexteer',NxtrConf,char(169),first,last)
      | end
  Enumerated Constant : simulink/Sources/Enumerated Constant  RequirementInfo="{'linktype_rmi_doors' '0000bb40 (/E-STEER Core/SubSystem Specifications/Application Functions/SF99/SF101A Motor Quadrant Detection)' '#SF101A_58' 'true' 'REQ:  SF101A_58' '' } %GIDa_d925bcc7_5572_4acd_aaab_a8684cfce636"  OutDataTypeStr=Enum: MotQuad1  Value=MotQuad1.MOTQUAD_QUAD1  SampleTime=inf
  Enumerated Constant1 : simulink/Sources/Enumerated Constant  RequirementInfo="{'linktype_rmi_doors' '0000bb40 (/E-STEER Core/SubSystem Specifications/Application Functions/SF99/SF101A Motor Quadrant Detection)' '#SF101A_58' 'true' 'REQ:  SF101A_58' '' } %GIDa_5030d704_8aea_4677_8253_42f3de2310d4"  OutDataTypeStr=Enum: MotQuad1  Value=MotQuad1.MOTQUAD_QUAD3  SampleTime=inf
  If : If  IfExpression=u1 ==1
  If Action Subsystem : Subsystem  TreatAsAtomicUnit=on
      settings: RTWSystemCode=Inline
  If Action Subsystem1 : Subsystem  TreatAsAtomicUnit=on
      settings: RTWSystemCode=Inline
  Merge : Merge
  Relational Operator : RelationalOperator  Operator===  OutDataTypeStr=boolean
  Out1 : Outport
  wires:
  In1/1 -> Relational Operator/1
  Constant/1 -> Relational Operator/2
  Relational Operator/1 -> If/1
  If/1 -> If Action Subsystem/Action
  If/2 -> If Action Subsystem1/Action
  If Action Subsystem/1(Out1) -> Merge/1
  If Action Subsystem1/1(Out1) -> Merge/2
  Merge/1 -> Out1/1
  Enumerated Constant/1 -> If Action Subsystem/1(In1)
  Enumerated Constant1/1 -> If Action Subsystem1/1(In1)

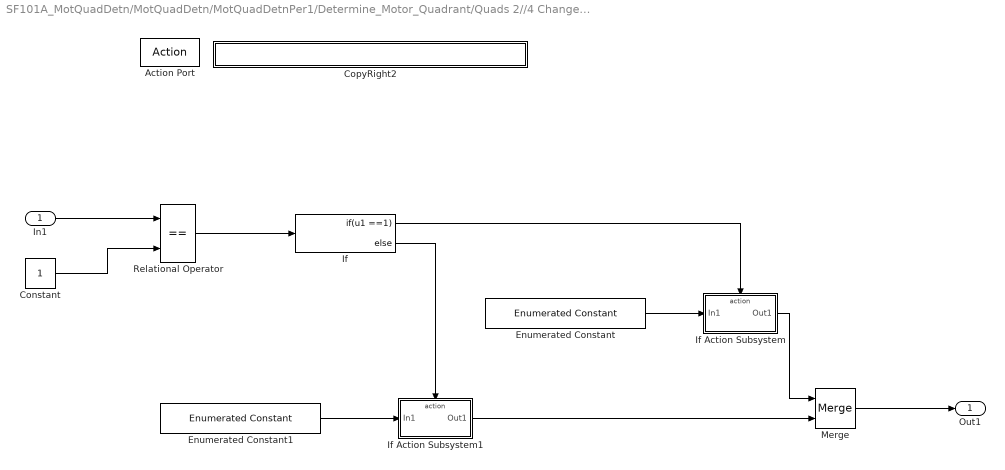
== system SF101A_MotQuadDetn/MotQuadDetn/MotQuadDetnPer1/Determine_Motor_Quadrant/Quads 2//4 Change in direction ==
  In1 : Inport
  Action Port : ActionPort  ActionType=else
  Constant : Constant  OutDataTypeStr=single
  CopyRight2 : Subsystem  Description=|  mask(Copyright Information){none=on}
      | Copyright info block.                                               
      |                                                                     
      | Place copyright information at the top of every subsystem in design.
      mask prompts: none "No parameters"
      mask help: Place copyright information at the top of every subsystem in design.
      mask Display:
      | NxtrConf = 'Nexteer Confidential';
      | 
      | sys = bdroot; %handle for the current model ("system")
      | first = get_param(sys,'Created');
      | if(isempty(first))
      |     first = datestr(now,'yyyy');
      | else
      |     first = first(end-3:end);  %year is last four digits
      | end
      | 
      | last = get_param(sys,'LastModifiedDate');
      | if isempty(last)
      |     last = datestr(now,'yyyy');
      | else
      |     last = last(end-3:end);
      | end
      | 
      | if strcmp(first,last)
      |     fprintf('%s -- Copyright %s Nexteer',NxtrConf,first)
      | else
      |     fprintf('%s -- %s%s- %s Nexteer',NxtrConf,char(169),first,last)
      | end
  Enumerated Constant : simulink/Sources/Enumerated Constant  RequirementInfo="{'linktype_rmi_doors' '0000bb40 (/E-STEER Core/SubSystem Specifications/Application Functions/SF99/SF101A Motor Quadrant Detection)' '#SF101A_58' 'true' 'REQ:  SF101A_58' '' } %GIDa_114bdeff_03c1_42d9_8d38_ef969e33a237"  OutDataTypeStr=Enum: MotQuad1  Value=MotQuad1.MOTQUAD_QUAD2  SampleTime=inf
  Enumerated Constant1 : simulink/Sources/Enumerated Constant  RequirementInfo="{'linktype_rmi_doors' '0000bb40 (/E-STEER Core/SubSystem Specifications/Application Functions/SF99/SF101A Motor Quadrant Detection)' '#SF101A_58' 'true' 'REQ:  SF101A_58' '' } %GIDa_62c46b86_0e1f_427f_a6f0_3d3bff6792a5"  OutDataTypeStr=Enum: MotQuad1  Value=MotQuad1.MOTQUAD_QUAD4  SampleTime=inf
  If : If  IfExpression=u1 ==1
  If Action Subsystem : Subsystem  TreatAsAtomicUnit=on
      settings: RTWSystemCode=Inline
  If Action Subsystem1 : Subsystem  TreatAsAtomicUnit=on
      settings: RTWSystemCode=Inline
  Merge : Merge
  Relational Operator : RelationalOperator  Operator===  OutDataTypeStr=boolean
  Out1 : Outport
  wires:
  Merge/1 -> Out1/1
  If Action Subsystem1/1(Out1) -> Merge/2
  If Action Subsystem/1(Out1) -> Merge/1
  Enumerated Constant/1 -> If Action Subsystem/1(In1)
  If/2 -> If Action Subsystem1/Action
  If/1 -> If Action Subsystem/Action
  Relational Operator/1 -> If/1
  Constant/1 -> Relational Operator/2
  In1/1 -> Relational Operator/1
  Enumerated Constant1/1 -> If Action Subsystem1/1(In1)

== system SF101A_MotQuadDetn/MotQuadDetn/MotQuadDetnPer1/Determine_TqCmd_Sign/CopyRight2 ==

== system SF101A_MotQuadDetn/MotQuadDetn/MotQuadDetnPer1/Determine_TqCmd_Sign/Determine Motor Torque Command Sign ==
  TqCmd : Inport
  Action Port : ActionPort  ActionType=then
  CopyRight2 : Subsystem  Description=|  mask(Copyright Information){none=on}
      | Copyright info block.                                               
      |                                                                     
      | Place copyright information at the top of every subsystem in design.
      mask prompts: none "No parameters"
      mask help: Place copyright information at the top of every subsystem in design.
      mask Display:
      | NxtrConf = 'Nexteer Confidential';
      | 
      | sys = bdroot; %handle for the current model ("system")
      | first = get_param(sys,'Created');
      | if(isempty(first))
      |     first = datestr(now,'yyyy');
      | else
      |     first = first(end-3:end);  %year is last four digits
      | end
      | 
      | last = get_param(sys,'LastModifiedDate');
      | if isempty(last)
      |     last = datestr(now,'yyyy');
      | else
      |     last = last(end-3:end);
      | end
      | 
      | if strcmp(first,last)
      |     fprintf('%s -- Copyright %s Nexteer',NxtrConf,first)
      | else
      |     fprintf('%s -- %s%s- %s Nexteer',NxtrConf,char(169),first,last)
      | end
  Sign_s08_f32 : NxtrSign/Sign_s08_f32  SFunctionSpec=int8 y1 = Sign_s08_f32(single u1)
  TqCmdSign : Outport
  wires:
  TqCmd/1 -> Sign_s08_f32/1
  Sign_s08_f32/1 -> TqCmdSign/1  "TqCmdSign"

== system SF101A_MotQuadDetn/MotQuadDetn/MotQuadDetnPer1/Determine_TqCmd_Sign/Determine Motor Torque Command Sign1 ==
  In1 : Inport
  Action Port : ActionPort  ActionType=else
  CopyRight2 : Subsystem  Description=|  mask(Copyright Information){none=on}
      | Copyright info block.                                               
      |                                                                     
      | Place copyright information at the top of every subsystem in design.
      mask prompts: none "No parameters"
      mask help: Place copyright information at the top of every subsystem in design.
      mask Display:
      | NxtrConf = 'Nexteer Confidential';
      | 
      | sys = bdroot; %handle for the current model ("system")
      | first = get_param(sys,'Created');
      | if(isempty(first))
      |     first = datestr(now,'yyyy');
      | else
      |     first = first(end-3:end);  %year is last four digits
      | end
      | 
      | last = get_param(sys,'LastModifiedDate');
      | if isempty(last)
      |     last = datestr(now,'yyyy');
      | else
      |     last = last(end-3:end);
      | end
      | 
      | if strcmp(first,last)
      |     fprintf('%s -- Copyright %s Nexteer',NxtrConf,first)
      | else
      |     fprintf('%s -- %s%s- %s Nexteer',NxtrConf,char(169),first,last)
      | end
  Out1 : Outport
  wires:
  In1/1 -> Out1/1

== system SF101A_MotQuadDetn/MotQuadDetn/MotQuadDetnPer1/Determine_Motor_Direction/If Action Subsystem/CopyRight2 ==

== system SF101A_MotQuadDetn/MotQuadDetn/MotQuadDetnPer1/Determine_Motor_Direction/If Action Subsystem1/CopyRight2 ==

== system SF101A_MotQuadDetn/MotQuadDetn/MotQuadDetnPer1/Determine_Motor_Direction/If Action Subsystem2/CopyRight2 ==

== system SF101A_MotQuadDetn/MotQuadDetn/MotQuadDetnPer1/Determine_Motor_Quadrant/Quads 1//3 No change in direction/CopyRight2 ==

== system SF101A_MotQuadDetn/MotQuadDetn/MotQuadDetnPer1/Determine_Motor_Quadrant/Quads 1//3 No change in direction/If Action Subsystem ==
  In1 : Inport
  Action Port : ActionPort  ActionType=then
  CopyRight2 : Subsystem  Description=|  mask(Copyright Information){none=on}
      | Copyright info block.                                               
      |                                                                     
      | Place copyright information at the top of every subsystem in design.
      mask prompts: none "No parameters"
      mask help: Place copyright information at the top of every subsystem in design.
      mask Display:
      | NxtrConf = 'Nexteer Confidential';
      | 
      | sys = bdroot; %handle for the current model ("system")
      | first = get_param(sys,'Created');
      | if(isempty(first))
      |     first = datestr(now,'yyyy');
      | else
      |     first = first(end-3:end);  %year is last four digits
      | end
      | 
      | last = get_param(sys,'LastModifiedDate');
      | if isempty(last)
      |     last = datestr(now,'yyyy');
      | else
      |     last = last(end-3:end);
      | end
      | 
      | if strcmp(first,last)
      |     fprintf('%s -- Copyright %s Nexteer',NxtrConf,first)
      | else
      |     fprintf('%s -- %s%s- %s Nexteer',NxtrConf,char(169),first,last)
      | end
  Out1 : Outport
  wires:
  In1/1 -> Out1/1

== system SF101A_MotQuadDetn/MotQuadDetn/MotQuadDetnPer1/Determine_Motor_Quadrant/Quads 1//3 No change in direction/If Action Subsystem1 ==
  In1 : Inport
  Action Port : ActionPort  ActionType=else
  CopyRight2 : Subsystem  Description=|  mask(Copyright Information){none=on}
      | Copyright info block.                                               
      |                                                                     
      | Place copyright information at the top of every subsystem in design.
      mask prompts: none "No parameters"
      mask help: Place copyright information at the top of every subsystem in design.
      mask Display:
      | NxtrConf = 'Nexteer Confidential';
      | 
      | sys = bdroot; %handle for the current model ("system")
      | first = get_param(sys,'Created');
      | if(isempty(first))
      |     first = datestr(now,'yyyy');
      | else
      |     first = first(end-3:end);  %year is last four digits
      | end
      | 
      | last = get_param(sys,'LastModifiedDate');
      | if isempty(last)
      |     last = datestr(now,'yyyy');
      | else
      |     last = last(end-3:end);
      | end
      | 
      | if strcmp(first,last)
      |     fprintf('%s -- Copyright %s Nexteer',NxtrConf,first)
      | else
      |     fprintf('%s -- %s%s- %s Nexteer',NxtrConf,char(169),first,last)
      | end
  Out1 : Outport
  wires:
  In1/1 -> Out1/1

== system SF101A_MotQuadDetn/MotQuadDetn/MotQuadDetnPer1/Determine_Motor_Quadrant/Quads 2//4 Change in direction/CopyRight2 ==

== system SF101A_MotQuadDetn/MotQuadDetn/MotQuadDetnPer1/Determine_Motor_Quadrant/Quads 2//4 Change in direction/If Action Subsystem ==
  In1 : Inport
  Action Port : ActionPort  ActionType=then
  CopyRight2 : Subsystem  Description=|  mask(Copyright Information){none=on}
      | Copyright info block.                                               
      |                                                                     
      | Place copyright information at the top of every subsystem in design.
      mask prompts: none "No parameters"
      mask help: Place copyright information at the top of every subsystem in design.
      mask Display:
      | NxtrConf = 'Nexteer Confidential';
      | 
      | sys = bdroot; %handle for the current model ("system")
      | first = get_param(sys,'Created');
      | if(isempty(first))
      |     first = datestr(now,'yyyy');
      | else
      |     first = first(end-3:end);  %year is last four digits
      | end
      | 
      | last = get_param(sys,'LastModifiedDate');
      | if isempty(last)
      |     last = datestr(now,'yyyy');
      | else
      |     last = last(end-3:end);
      | end
      | 
      | if strcmp(first,last)
      |     fprintf('%s -- Copyright %s Nexteer',NxtrConf,first)
      | else
      |     fprintf('%s -- %s%s- %s Nexteer',NxtrConf,char(169),first,last)
      | end
  Out1 : Outport
  wires:
  In1/1 -> Out1/1
